simulink model "PD_controller"  (R2021b)
settings: Solver=ode4  StartTime=0.0  StopTime=10.0  FixedStep=0.001  RelTol=1e-3
values from neighbouring files (symbols this model uses):
  Ki = 5    [mainPD.m]
  Kp = K_p(i)    [mainPD.m]
libraries: RCTblocks x1
settings Model: Creator=Mando  LastModifiedBy=Mando

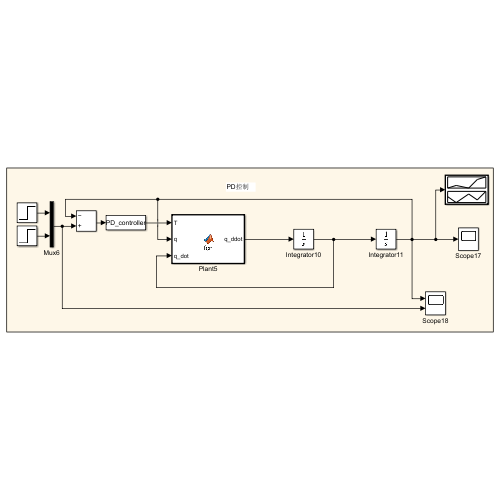
[thumbnail: Simulink's stored preview of the top-level diagram]
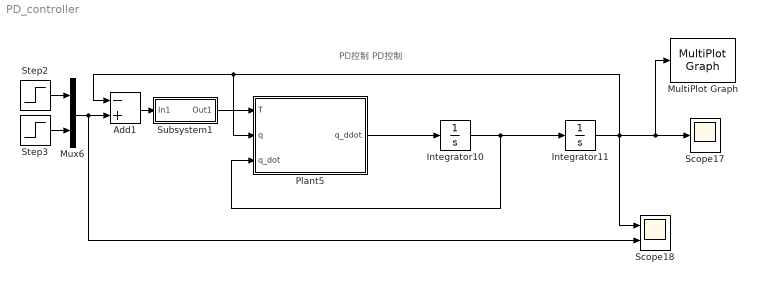
== system PD_controller ==
  note: PD控制
      | PD控制
  Add1 : Sum  Inputs=-+
  Integrator10 : Integrator  InitialCondition=[1; 1]
  Integrator11 : Integrator  InitialCondition=[0.5; 1]
  MultiPlot Graph : RCTblocks/MultiPlot Graph  Tag=MultiPlot  tmin=0  tmax=20  ymin=-1  ymax=1  Tsamp=-1  vnamesave=multisimout
      settings: SourceProductBaseCode=RC
  Mux6 : Mux  Inputs=2
  Plant5 : MATLAB Function  TreatAsAtomicUnit=on
  Scope17 : Scope
  Scope18 : Scope  NumInputPorts=2
  Step2 : Step  Time=0  SampleTime=0
  Step3 : Step  Time=0  SampleTime=0
  Subsystem1 : Subsystem
      mask Display: disp('PD_controller')
  wires:
  Plant5/1(q_ddot) -> Integrator10/1
  Integrator10/1 -> Integrator11/1, Plant5/3(q_dot)
  Integrator11/1 -> Plant5/2(q), Add1/1, MultiPlot Graph/1, Scope17/1, Scope18/1
  Mux6/1 -> Add1/2, Scope18/2
  Add1/1 -> Subsystem1/1(In1)
  Step2/1 -> Mux6/1
  Subsystem1/1(Out1) -> Plant5/1(T)
  Step3/1 -> Mux6/2

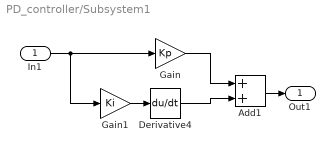
== system PD_controller/Subsystem1 ==
  In1 : Inport
  Add1 : Sum
  Derivative4 : Derivative
  Gain : Gain  Gain=Kp
  Gain1 : Gain  Gain=Ki
  Out1 : Outport
  wires:
  Derivative4/1 -> Add1/2
  Gain/1 -> Add1/1
  Add1/1 -> Out1/1
  In1/1 -> Gain/1, Gain1/1
  Gain1/1 -> Derivative4/1

== matlab function PD_controller/Plant5 ==
  data: T input; q_ddot output; q input; q_dot input
function q_ddot = fcn(T, q, q_dot)
%Defining given parameters
p1=2.9;
p2=0.76;
p3=0.87;
p4=3.04;
p5=0.87;
g=9.8;


%Defining Robot Dynamic Model
M = [p1+p2+2*p3*cos(q(2)),p2+p3*cos(q(2));p2+p3*cos(q(2)),p2];
Vm=[-p3*q_dot(2)*sin(q(2)) -p3*(q_dot(1)+q_dot(2))*sin(q(2)); p3*q_dot(1)*sin(q(2)) 0];
G= [p4*g*cos(q(1))+p5*g*cos(q(1)+q(2));p5*g*cos(q(1)+q(2))];

%Robot Dynamics
q_ddot = inv(M)*(T - (Vm*q_dot) - G);
